simulink model "SEA_NonLineare"  (R2013a)
settings: Solver=ode45  StartTime=0.0  StopTime=10.0  RelTol=1e-3
values from neighbouring files (symbols this model uses):
  b = 0.0575*Kg*m^2/rad    (= 0.0575)    [prova.m]
  d = 2.5185*Kg*m^2/(rad*s)    (= 2.5185)    [prova.m]
  g = 9.81*m/s^2    (= 9.81)    [prova.m]
  j = 0.2156*Kg*m^2/rad    (= 0.2156)    [prova.m]
  k = 200*Nm/rad    (= 200)    [prova.m]
  l = 0.5*m    (= 0.5)    [prova.m]
  M = 0.15*Kg    (= 0.15)    [prova.m]
  x0 = x_e+dx0    [prova.m]
settings Model: Creator=peppe  LastModifiedBy=peppe

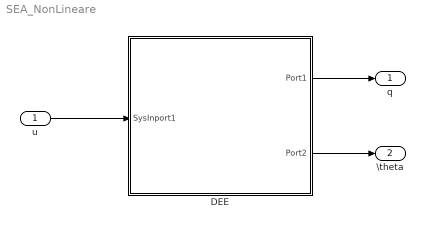
== system SEA_NonLineare ==
  u : Inport
  DEE : Subsystem  mask(Differential Equation Editor (DEE)){}
      settings: OpenFcn=diffeqed
      mask Display: disp('Differential Equation\n Editor')
  q : Outport
  \theta : Outport  Port=2
  wires:
  u/1 -> DEE/1(SysInport1)
  DEE/2(Port2) -> \theta/1
  DEE/1(Port1) -> q/1

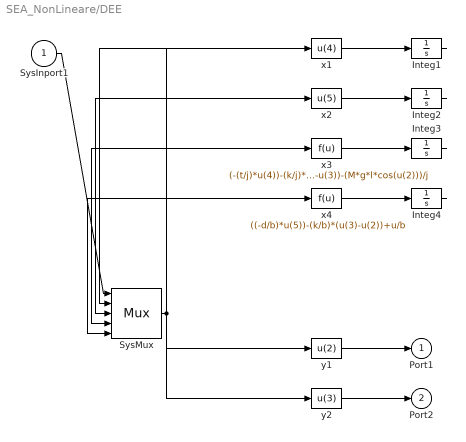
== system SEA_NonLineare/DEE ==
  SysInport1 : Inport
  Integ1 : Integrator  InitialCondition=x0(1)
  Integ2 : Integrator  InitialCondition=x0(2)
  Integ3 : Integrator  InitialCondition=x0(3)
  Integ4 : Integrator  InitialCondition=x0(4)
  SysMux : Mux  Inputs=5
  x1 : Fcn  Expr=u(4)
  x2 : Fcn  Expr=u(5)
  x3 : Fcn  Expr=(-(t/j)*u(4))-(k/j)*(u(2)-u(3))-(M*g*l*cos(u(2)))/j
  x4 : Fcn  Expr=((-d/b)*u(5))-(k/b)*(u(3)-u(2))+u/b
  y1 : Fcn  Expr=u(2)
  y2 : Fcn  Expr=u(3)
  Port1 : Outport
  Port2 : Outport  Port=2
  wires:
  SysInport1/1 -> SysMux/1
  SysMux/1 -> x1/1, x2/1, x3/1, x4/1, y1/1, y2/1
  x1/1 -> Integ1/1
  Integ1/1 -> SysMux/2
  x2/1 -> Integ2/1
  Integ2/1 -> SysMux/3
  x3/1 -> Integ3/1
  Integ3/1 -> SysMux/4
  x4/1 -> Integ4/1
  Integ4/1 -> SysMux/5
  y1/1 -> Port1/1
  y2/1 -> Port2/1
